simulink library "SG_library"  (R2022b)
settings: Solver=VariableStepAuto  StartTime=0.0  StopTime=10.0  RelTol=1e-3
undefined symbols (not defined in the file or in its folder): a, b, c, dfilt, GeneratorType, IO324, IO324_FPGA, IO324_src, IO334, IO334_FPGA, IO334_src, IO397, IO397_FPGA, IO397_src, repelem
libraries: speedgoatlib_hdlCoder_IO3xx x44, $bdroot x11, slrealtimeutilitieslib x9, simulink x6, hdlsllib x6, dspsrcs4 x2, dsparch4 x2
(part 2 of 3)

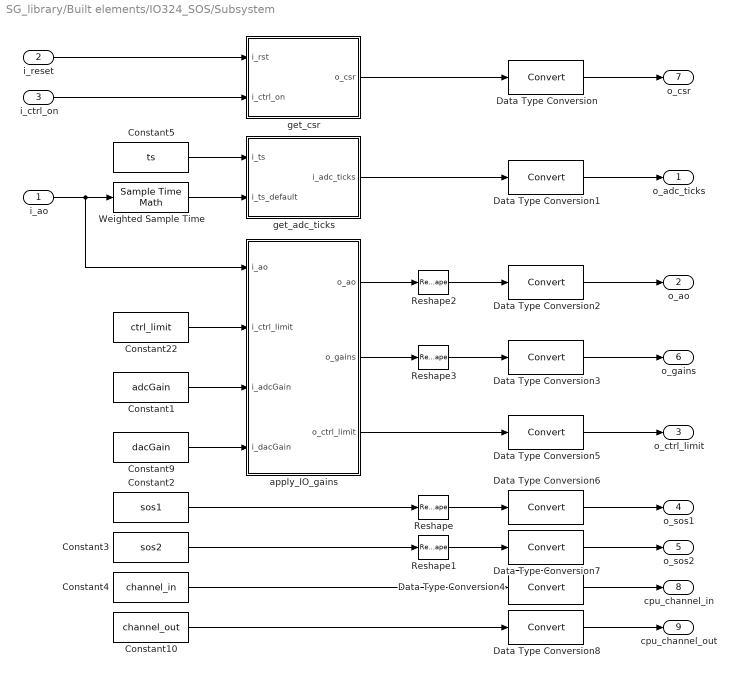
== system SG_library/Built elements/IO324_SOS/Subsystem ==
  i_ao : Inport
  i_reset : Inport  Port=2
  i_ctrl_on : Inport  Port=3
  Constant1 : Constant  Value=adcGain  SampleTime=-1
  Constant10 : Constant  Value=channel_out  SampleTime=-1
  Constant2 : Constant  Value=sos1  SampleTime=-1
  Constant22 : Constant  Value=ctrl_limit  SampleTime=-1
  Constant3 : Constant  Value=sos2  SampleTime=-1
  Constant4 : Constant  Value=channel_in  SampleTime=-1
  Constant5 : Constant  Value=ts  SampleTime=-1
  Constant9 : Constant  Value=dacGain  SampleTime=-1
  Data Type Conversion{,1..8} (9 alike) : DataTypeConversion  SaturateOnIntegerOverflow=off  RndMeth=Floor
  Reshape{,1..3} (4 alike) : Reshape
  Weighted Sample Time : SampleTimeMath  TsampMathOp=Ts Only
  apply_IO_gains : MATLAB Function  TreatAsAtomicUnit=on
  get_adc_ticks : MATLAB Function  TreatAsAtomicUnit=on
  get_csr : MATLAB Function  TreatAsAtomicUnit=on
  o_adc_ticks : Outport
  o_ao : Outport  Port=2
  o_ctrl_limit : Outport  Port=3
  o_sos1 : Outport  Port=4
  o_sos2 : Outport  Port=5
  o_gains : Outport  Port=6
  o_csr : Outport  Port=7
  cpu_channel_in : Outport  Port=8
  cpu_channel_out : Outport  Port=9
  wires:
  i_reset/1 -> get_csr/1(i_rst)
  i_ctrl_on/1 -> get_csr/2(i_ctrl_on)
  Constant5/1 -> get_adc_ticks/1(i_ts)
  Weighted Sample Time/1 -> get_adc_ticks/2(i_ts_default)
  i_ao/1 -> apply_IO_gains/1(i_ao), Weighted Sample Time/1
  get_adc_ticks/1(i_adc_ticks) -> Data Type Conversion1/1
  Constant1/1 -> apply_IO_gains/3(i_adcGain)
  Constant9/1 -> apply_IO_gains/4(i_dacGain)
  Constant22/1 -> apply_IO_gains/2(i_ctrl_limit)
  get_csr/1(o_csr) -> Data Type Conversion/1
  Constant2/1 -> Reshape/1
  Constant3/1 -> Reshape1/1
  Data Type Conversion/1 -> o_csr/1
  Data Type Conversion1/1 -> o_adc_ticks/1
  Data Type Conversion2/1 -> o_ao/1
  Data Type Conversion3/1 -> o_gains/1
  Data Type Conversion5/1 -> o_ctrl_limit/1
  Data Type Conversion6/1 -> o_sos1/1
  Data Type Conversion7/1 -> o_sos2/1
  Reshape/1 -> Data Type Conversion6/1
  Reshape1/1 -> Data Type Conversion7/1
  apply_IO_gains/3(o_ctrl_limit) -> Data Type Conversion5/1
  apply_IO_gains/2(o_gains) -> Reshape3/1
  apply_IO_gains/1(o_ao) -> Reshape2/1
  Reshape2/1 -> Data Type Conversion2/1
  Reshape3/1 -> Data Type Conversion3/1
  Data Type Conversion4/1 -> cpu_channel_in/1
  Constant10/1 -> Data Type Conversion8/1
  Constant4/1 -> Data Type Conversion4/1
  Data Type Conversion8/1 -> cpu_channel_out/1

== system SG_library/Built elements/IO324_SOS/Subsystem1 ==
  i_ai : Inport
  i_ao_monitor : Inport  Port=2
  i_staurated : Inport  Port=3
  Constant1 : Constant  Value=adcGain  SampleTime=-1
  Constant9 : Constant  Value=dacGain  SampleTime=-1
  Data Type Conversion : DataTypeConversion  OutDataTypeStr=double  SaturateOnIntegerOverflow=off  RndMeth=Floor
  Data Type Conversion1 : DataTypeConversion  OutDataTypeStr=double  SaturateOnIntegerOverflow=off  RndMeth=Floor
  Reshape : Reshape
  apply_IO_gains : MATLAB Function  TreatAsAtomicUnit=on
  o_ai : Outport
  o_ao_monitor : Outport  Port=2
  o_saturated : Outport  Port=3
  wires:
  Constant9/1 -> apply_IO_gains/4(i_dacGain)
  apply_IO_gains/1(o_ai) -> Reshape/1
  Constant1/1 -> apply_IO_gains/3(i_adcGain)
  i_ai/1 -> Data Type Conversion/1
  i_ao_monitor/1 -> Data Type Conversion1/1
  Reshape/1 -> o_ai/1
  apply_IO_gains/2(o_ao_monitor) -> o_ao_monitor/1
  Data Type Conversion1/1 -> apply_IO_gains/2(i_ao_monitor)
  Data Type Conversion/1 -> apply_IO_gains/1(i_ai)
  i_staurated/1 -> o_saturated/1

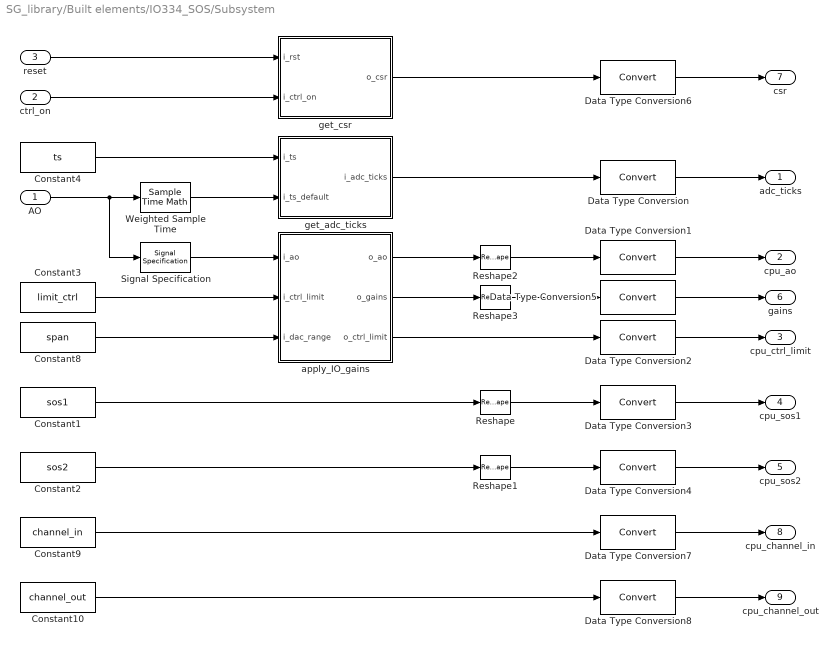
== system SG_library/Built elements/IO334_SOS/Subsystem ==
  AO : Inport
  ctrl_on : Inport  Port=2
  reset : Inport  Port=3
  Constant1 : Constant  Value=sos1  SampleTime=-1
  Constant10 : Constant  Value=channel_out  SampleTime=-1
  Constant2 : Constant  Value=sos2  SampleTime=-1
  Constant3 : Constant  Value=limit_ctrl  SampleTime=-1
  Constant4 : Constant  Value=ts  SampleTime=-1
  Constant8 : Constant  Value=span  SampleTime=-1
  Constant9 : Constant  Value=channel_in  SampleTime=-1
  Data Type Conversion{,1..8} (9 alike) : DataTypeConversion  SaturateOnIntegerOverflow=off  RndMeth=Floor
  Reshape{,1..3} (4 alike) : Reshape
  Signal Specification : SignalSpecification  Dimensions=16
  Weighted Sample Time : SampleTimeMath  TsampMathOp=Ts Only
  apply_IO_gains : MATLAB Function  TreatAsAtomicUnit=on
  get_adc_ticks : MATLAB Function  TreatAsAtomicUnit=on
  get_csr : MATLAB Function  TreatAsAtomicUnit=on
  adc_ticks : Outport
  cpu_ao : Outport  Port=2
  cpu_ctrl_limit : Outport  Port=3
  cpu_sos1 : Outport  Port=4
  cpu_sos2 : Outport  Port=5
  gains : Outport  Port=6
  csr : Outport  Port=7
  cpu_channel_in : Outport  Port=8
  cpu_channel_out : Outport  Port=9
  wires:
  Constant3/1 -> apply_IO_gains/2(i_ctrl_limit)
  apply_IO_gains/1(o_ao) -> Reshape2/1
  apply_IO_gains/3(o_ctrl_limit) -> Data Type Conversion2/1
  apply_IO_gains/2(o_gains) -> Reshape3/1
  get_adc_ticks/1(i_adc_ticks) -> Data Type Conversion/1
  Weighted Sample Time/1 -> get_adc_ticks/2(i_ts_default)
  Constant4/1 -> get_adc_ticks/1(i_ts)
  get_csr/1(o_csr) -> Data Type Conversion6/1
  ctrl_on/1 -> get_csr/2(i_ctrl_on)
  reset/1 -> get_csr/1(i_rst)
  Data Type Conversion6/1 -> csr/1
  Data Type Conversion5/1 -> gains/1
  Data Type Conversion4/1 -> cpu_sos2/1
  Data Type Conversion3/1 -> cpu_sos1/1
  Data Type Conversion2/1 -> cpu_ctrl_limit/1
  Data Type Conversion1/1 -> cpu_ao/1
  Data Type Conversion/1 -> adc_ticks/1
  Reshape1/1 -> Data Type Conversion4/1
  Reshape/1 -> Data Type Conversion3/1
  Constant8/1 -> apply_IO_gains/3(i_dac_range)
  Signal Specification/1 -> apply_IO_gains/1(i_ao)
  Constant1/1 -> Reshape/1
  AO/1 -> Signal Specification/1, Weighted Sample Time/1
  Constant2/1 -> Reshape1/1
  Reshape2/1 -> Data Type Conversion1/1
  Reshape3/1 -> Data Type Conversion5/1
  Constant10/1 -> Data Type Conversion8/1
  Constant9/1 -> Data Type Conversion7/1
  Data Type Conversion7/1 -> cpu_channel_in/1
  Data Type Conversion8/1 -> cpu_channel_out/1

== system SG_library/Built elements/IO334_SOS/Subsystem1 ==
  i_ai : Inport
  i_monitor : Inport  Port=2
  i_staurated : Inport  Port=3
  Constant : Constant  Value=span  SampleTime=-1
  Data Type Conversion : DataTypeConversion  OutDataTypeStr=double  SaturateOnIntegerOverflow=off  RndMeth=Floor
  Data Type Conversion1 : DataTypeConversion  OutDataTypeStr=double  SaturateOnIntegerOverflow=off  RndMeth=Floor
  Reshape : Reshape
  apply_IO_gains : MATLAB Function  TreatAsAtomicUnit=on
  o_ai : Outport
  o_monitor : Outport  Port=2
  o_saturated : Outport  Port=3
  wires:
  apply_IO_gains/1(o_ai) -> Reshape/1
  Constant/1 -> apply_IO_gains/3(i_dac_span)
  i_ai/1 -> Data Type Conversion/1
  i_monitor/1 -> Data Type Conversion1/1
  Reshape/1 -> o_ai/1
  apply_IO_gains/2(o_ao_monitor) -> o_monitor/1
  Data Type Conversion/1 -> apply_IO_gains/1(i_ai)
  Data Type Conversion1/1 -> apply_IO_gains/2(i_ao_monitor)
  i_staurated/1 -> o_saturated/1

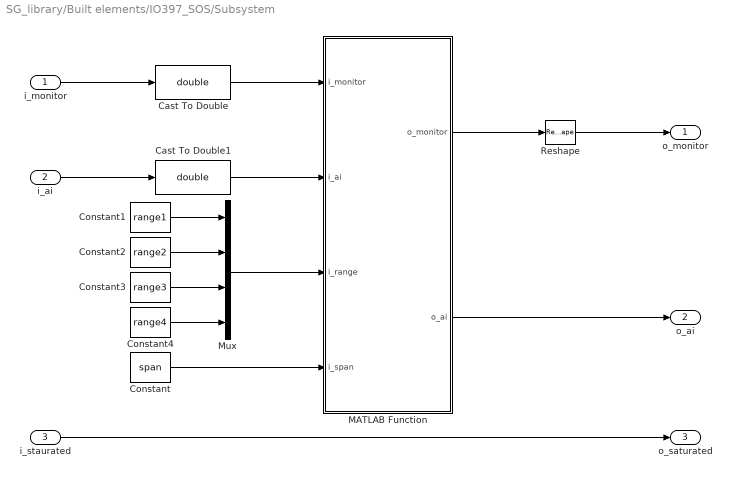
== system SG_library/Built elements/IO397_SOS/Subsystem ==
  i_monitor : Inport
  i_ai : Inport  Port=2
  i_staurated : Inport  Port=3
  Cast To Double : DataTypeConversion  OutDataTypeStr=double  SaturateOnIntegerOverflow=off  RndMeth=Floor
  Cast To Double1 : DataTypeConversion  OutDataTypeStr=double  SaturateOnIntegerOverflow=off  RndMeth=Floor
  Constant : Constant  Value=span  SampleTime=-1
  Constant1 : Constant  Value=range1  SampleTime=-1
  Constant2 : Constant  Value=range2  SampleTime=-1
  Constant3 : Constant  Value=range3  SampleTime=-1
  Constant4 : Constant  Value=range4  SampleTime=-1
  MATLAB Function : MATLAB Function  TreatAsAtomicUnit=on
  Mux : Mux
  Reshape : Reshape
  o_monitor : Outport
  o_ai : Outport  Port=2
  o_saturated : Outport  Port=3
  wires:
  Constant3/1 -> Mux/3
  Constant1/1 -> Mux/1
  MATLAB Function/1(o_monitor) -> Reshape/1
  Constant/1 -> MATLAB Function/4(i_span)
  Constant2/1 -> Mux/2
  Mux/1 -> MATLAB Function/3(i_range)
  Constant4/1 -> Mux/4
  MATLAB Function/2(o_ai) -> o_ai/1
  i_monitor/1 -> Cast To Double/1
  i_ai/1 -> Cast To Double1/1
  Reshape/1 -> o_monitor/1
  Cast To Double/1 -> MATLAB Function/1(i_monitor)
  Cast To Double1/1 -> MATLAB Function/2(i_ai)
  i_staurated/1 -> o_saturated/1

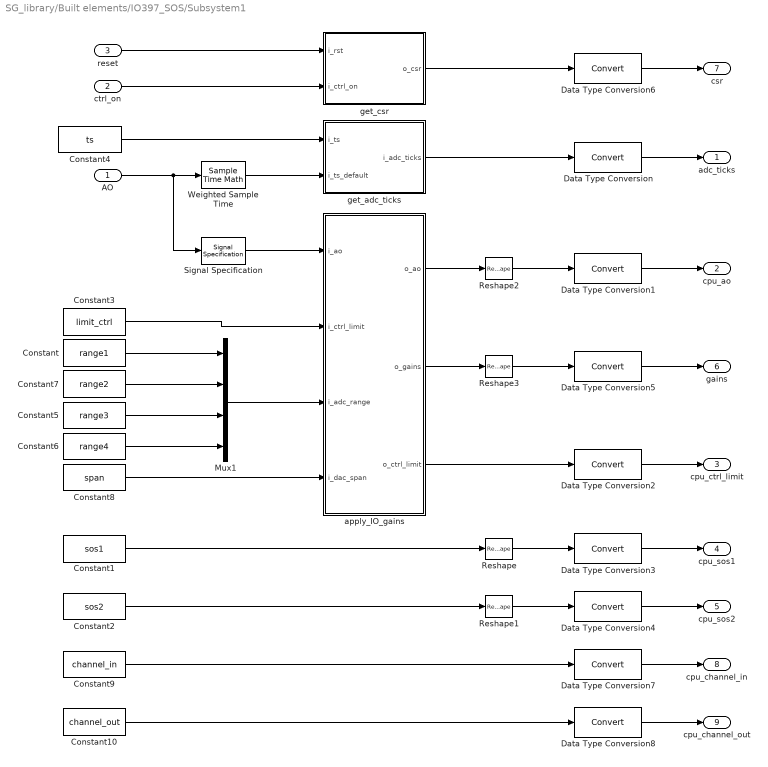
== system SG_library/Built elements/IO397_SOS/Subsystem1 ==
  AO : Inport
  ctrl_on : Inport  Port=2
  reset : Inport  Port=3
  Constant : Constant  Value=range1  SampleTime=-1
  Constant1 : Constant  Value=sos1  SampleTime=-1
  Constant10 : Constant  Value=channel_out  SampleTime=-1
  Constant2 : Constant  Value=sos2  SampleTime=-1
  Constant3 : Constant  Value=limit_ctrl  SampleTime=-1
  Constant4 : Constant  Value=ts  SampleTime=-1
  Constant5 : Constant  Value=range3  SampleTime=-1
  Constant6 : Constant  Value=range4  SampleTime=-1
  Constant7 : Constant  Value=range2  SampleTime=-1
  Constant8 : Constant  Value=span  SampleTime=-1
  Constant9 : Constant  Value=channel_in  SampleTime=-1
  Data Type Conversion{,1..8} (9 alike) : DataTypeConversion  SaturateOnIntegerOverflow=off  RndMeth=Floor
  Mux1 : Mux
  Reshape{,1..3} (4 alike) : Reshape
  Signal Specification : SignalSpecification  Dimensions=4
  Weighted Sample Time : SampleTimeMath  TsampMathOp=Ts Only
  apply_IO_gains : MATLAB Function  TreatAsAtomicUnit=on
  get_adc_ticks : MATLAB Function  TreatAsAtomicUnit=on
  get_csr : MATLAB Function  TreatAsAtomicUnit=on
  adc_ticks : Outport
  cpu_ao : Outport  Port=2
  cpu_ctrl_limit : Outport  Port=3
  cpu_sos1 : Outport  Port=4
  cpu_sos2 : Outport  Port=5
  gains : Outport  Port=6
  csr : Outport  Port=7
  cpu_channel_in : Outport  Port=8
  cpu_channel_out : Outport  Port=9
  wires:
  Constant2/1 -> Reshape1/1
  AO/1 -> Weighted Sample Time/1, Signal Specification/1
  Constant1/1 -> Reshape/1
  Constant7/1 -> Mux1/2
  Signal Specification/1 -> apply_IO_gains/1(i_ao)
  Constant/1 -> Mux1/1
  Mux1/1 -> apply_IO_gains/3(i_adc_range)
  Constant5/1 -> Mux1/3
  Constant6/1 -> Mux1/4
  Constant8/1 -> apply_IO_gains/4(i_dac_span)
  Reshape/1 -> Data Type Conversion3/1
  Reshape1/1 -> Data Type Conversion4/1
  Data Type Conversion/1 -> adc_ticks/1
  Data Type Conversion1/1 -> cpu_ao/1
  Data Type Conversion2/1 -> cpu_ctrl_limit/1
  Data Type Conversion3/1 -> cpu_sos1/1
  Data Type Conversion4/1 -> cpu_sos2/1
  Data Type Conversion5/1 -> gains/1
  Data Type Conversion6/1 -> csr/1
  reset/1 -> get_csr/1(i_rst)
  ctrl_on/1 -> get_csr/2(i_ctrl_on)
  get_csr/1(o_csr) -> Data Type Conversion6/1
  Constant4/1 -> get_adc_ticks/1(i_ts)
  Weighted Sample Time/1 -> get_adc_ticks/2(i_ts_default)
  get_adc_ticks/1(i_adc_ticks) -> Data Type Conversion/1
  apply_IO_gains/2(o_gains) -> Reshape3/1
  apply_IO_gains/1(o_ao) -> Reshape2/1
  Constant3/1 -> apply_IO_gains/2(i_ctrl_limit)
  Reshape2/1 -> Data Type Conversion1/1
  Reshape3/1 -> Data Type Conversion5/1
  apply_IO_gains/3(o_ctrl_limit) -> Data Type Conversion2/1
  Data Type Conversion7/1 -> cpu_channel_in/1
  Data Type Conversion8/1 -> cpu_channel_out/1
  Constant9/1 -> Data Type Conversion7/1
  Constant10/1 -> Data Type Conversion8/1

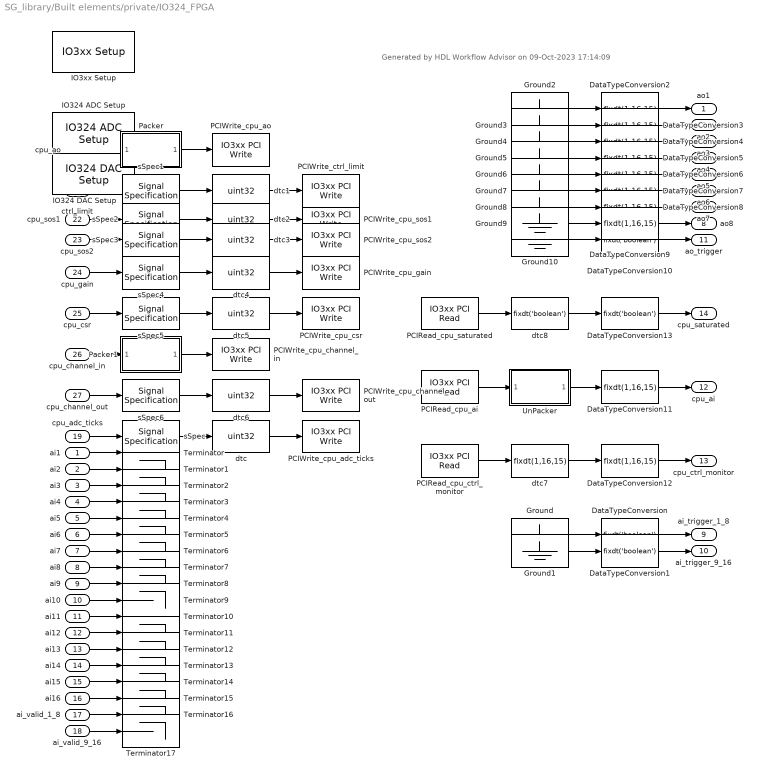
== system SG_library/Built elements/private/IO324_FPGA ==
  note: Generated by HDL Workflow Advisor on 09-Oct-2023 17:14:09
  ai1 : Inport  OutDataTypeStr=fixdt(1,16,15)
  ai2 : Inport  Port=2  OutDataTypeStr=fixdt(1,16,15)
  ai3 : Inport  Port=3  OutDataTypeStr=fixdt(1,16,15)
  ai4 : Inport  Port=4  OutDataTypeStr=fixdt(1,16,15)
  ai5 : Inport  Port=5  OutDataTypeStr=fixdt(1,16,15)
  ai6 : Inport  Port=6  OutDataTypeStr=fixdt(1,16,15)
  ai7 : Inport  Port=7  OutDataTypeStr=fixdt(1,16,15)
  ai8 : Inport  Port=8  OutDataTypeStr=fixdt(1,16,15)
  ai9 : Inport  Port=9  OutDataTypeStr=fixdt(1,16,15)
  ai10 : Inport  Port=10  OutDataTypeStr=fixdt(1,16,15)
  ai11 : Inport  Port=11  OutDataTypeStr=fixdt(1,16,15)
  ai12 : Inport  Port=12  OutDataTypeStr=fixdt(1,16,15)
  ai13 : Inport  Port=13  OutDataTypeStr=fixdt(1,16,15)
  ai14 : Inport  Port=14  OutDataTypeStr=fixdt(1,16,15)
  ai15 : Inport  Port=15  OutDataTypeStr=fixdt(1,16,15)
  ai16 : Inport  Port=16  OutDataTypeStr=fixdt(1,16,15)
  ai_valid_1_8 : Inport  Port=17  OutDataTypeStr=boolean
  ai_valid_9_16 : Inport  Port=18  OutDataTypeStr=boolean
  cpu_adc_ticks : Inport  Port=19  OutDataTypeStr=uint32
  cpu_ao : Inport  Port=20  OutDataTypeStr=fixdt(1,16,15)
  ctrl_limit : Inport  Port=21  OutDataTypeStr=fixdt(1,16,15)
  cpu_sos1 : Inport  Port=22  OutDataTypeStr=fixdt(1,32,26)
  cpu_sos2 : Inport  Port=23  OutDataTypeStr=fixdt(1,32,26)
  cpu_gain : Inport  Port=24  OutDataTypeStr=fixdt(1,32,16)
  cpu_csr : Inport  Port=25  OutDataTypeStr=uint8
  cpu_channel_in : Inport  Port=26
  cpu_channel_out : Inport  Port=27
  DataTypeConversion{,1,10,13} (4 alike) : DataTypeConversion  OutDataTypeStr=fixdt('boolean')  ConvertRealWorld=Stored Integer (SI)  SaturateOnIntegerOverflow=off  RndMeth=Floor
  DataTypeConversion{2..9,11..12} (10 alike) : DataTypeConversion  OutDataTypeStr=fixdt(1,16,15)  ConvertRealWorld=Stored Integer (SI)  SaturateOnIntegerOverflow=off  RndMeth=Floor
  Ground{,1..10} (11 alike) : Ground
  IO324 ADC Setup : speedgoatlib_hdlCoder_IO3xx/IO324 ADC Setup  module_id=module_id  adcGain_1=10.24V  adcActiv_1=on  adcDiffSelect_1=off  adcGain_2=10.24V  adcActiv_2=on  adcDiffSelect_2=off  adcGain_3=10.24V  adcActiv_3=on  adcDiffSelect_3=off  adcGain_4=10.24V  adcActiv_4=on  adcDiffSelect_4=off  adcGain_5=10.24V  adcActiv_5=on  adcDiffSelect_5=off  adcGain_6=10.24V  adcActiv_6=on  adcDiffSelect_6=off  adcGain_7=10.24V  adcActiv_7=on  adcDiffSelect_7=off  adcGain_8=10.24V  adcActiv_8=on  adcDiffSelect_8=off  adcGain_9=10.24V  adcActiv_9=on  adcDiffSelect_9=off  adcGain_10=10.24V  adcActiv_10=on  adcDiffSelect_10=off  adcGain_11=10.24V  adcActiv_11=on  adcDiffSelect_11=off  adcGain_12=10.24V  adcActiv_12=on  adcDiffSelect_12=off  adcGain_13=10.24V  adcActiv_13=on  adcDiffSelect_13=off  adcGain_14=10.24V  adcActiv_14=on  adcDiffSelect_14=off  adcGain_15=10.24V  adcActiv_15=on  adcDiffSelect_15=off  adcGain_16=10.24V  adcActiv_16=on  adcDiffSelect_16=off  adcGain_17=10.24V  adcActiv_17=off  adcDiffSelect_17=off  adcGain_18=10.24V  adcActiv_18=off  adcDiffSelect_18=off  adcGain_19=10.24V  adcActiv_19=off  adcDiffSelect_19=off  adcGain_20=10.24V  adcActiv_20=off  adcDiffSelect_20=off  adcGain_21=10.24V  adcActiv_21=off  adcDiffSelect_21=off  adcGain_22=10.24V  adcActiv_22=off  adcDiffSelect_22=off  adcGain_23=10.24V  adcActiv_23=off  adcDiffSelect_23=off  adcGain_24=10.24V  adcActiv_24=off  adcDiffSelect_24=off  adcGain_25=10.24V  adcActiv_25=off  adcDiffSelect_25=off  adcGain_26=10.24V  adcActiv_26=off  adcDiffSelect_26=off  adcGain_27=10.24V  adcActiv_27=off  adcDiffSelect_27=off  adcGain_28=10.24V  adcActiv_28=off  adcDiffSelect_28=off  adcGain_29=10.24V  adcActiv_29=off  adcDiffSelect_29=off  adcGain_30=10.24V  adcActiv_30=off  adcDiffSelect_30=off  adcGain_31=10.24V  adcActiv_31=off  adcDiffSelect_31=off  adcGain_32=10.24V  adcActiv_32=off  adcDiffSelect_32=off
  IO324 DAC Setup : speedgoatlib_hdlCoder_IO3xx/IO324 DAC Setup  module_id=module_id  dacGain_1=10.0V  dacActiv_1=on  dacGain_2=10.0V  dacActiv_2=on  dacGain_3=10.0V  dacActiv_3=on  dacGain_4=10.0V  dacActiv_4=on  dacGain_5=10.0V  dacActiv_5=on  dacGain_6=10.0V  dacActiv_6=on  dacGain_7=10.0V  dacActiv_7=on  dacGain_8=10.0V  dacActiv_8=on
  IO3xx Setup : speedgoatlib_hdlCoder_IO3xx/IO3xx Setup  mdl_ss_name=IO324_src/IO324_FPGA  board_type=IO324-200k  fpga_sync_mode=on  reset_mode=on  reset_mode_stop=on  device_id=1  module_id=module_id  pci_slot=slot  fpga_mat_file=C:\Speedgoat\Build\IO324_SOS\hdlsrc\IO324_src\IO324_FPGA.mat  timestamp_mcs=10/09/23 17:11:49  timestamp=2310091624  tsreg=hex2dec('8')  bsf_file=IO324_FPGA_2310091624.mcs  mcs=0  device_tree_overlays=Test.dtbo  init_reg_list=[]
  PCIRead_cpu_ai : speedgoatlib_hdlCoder_IO3xx/IO3xx PCI Read  device_id=1  module_id=module_id  board_type=IO324-200k  port_name=cpu_ai  port_offset=hex2dec('220')  port_type=uint32  port_dim=8  strobe=hex2dec('240')  sample_time=ts
  PCIRead_cpu_ctrl_monitor : speedgoatlib_hdlCoder_IO3xx/IO3xx PCI Read  device_id=1  module_id=module_id  board_type=IO324-200k  port_name=cpu_ctrl_monitor  port_offset=hex2dec('120')  port_type=uint32  port_dim=1  strobe=0  sample_time=ts
  PCIRead_cpu_saturated : speedgoatlib_hdlCoder_IO3xx/IO3xx PCI Read  device_id=1  module_id=module_id  board_type=IO324-200k  port_name=cpu_saturated  port_offset=hex2dec('124')  port_type=uint32  port_dim=1  strobe=0  sample_time=ts
  PCIWrite_cpu_adc_ticks : speedgoatlib_hdlCoder_IO3xx/IO3xx PCI Write  device_id=1  module_id=module_id  board_type=IO324-200k  port_name=cpu_adc_ticks  port_offset=hex2dec('100')  port_type=uint32  port_dim=1  strobe=0  sample_time=ts
  PCIWrite_cpu_ao : speedgoatlib_hdlCoder_IO3xx/IO3xx PCI Write  device_id=1  module_id=module_id  board_type=IO324-200k  port_name=cpu_ao  port_offset=hex2dec('130')  port_type=uint32  port_dim=4  strobe=hex2dec('140')  sample_time=ts
  PCIWrite_cpu_channel_in : speedgoatlib_hdlCoder_IO3xx/IO3xx PCI Write  device_id=1  module_id=module_id  board_type=IO324-200k  port_name=cpu_channel_in  port_offset=hex2dec('118')  port_type=uint32  port_dim=1  strobe=0  sample_time=ts
  PCIWrite_cpu_channel_out : speedgoatlib_hdlCoder_IO3xx/IO3xx PCI Write  device_id=1  module_id=module_id  board_type=IO324-200k  port_name=cpu_channel_out  port_offset=hex2dec('11C')  port_type=uint32  port_dim=1  strobe=0  sample_time=ts
  PCIWrite_cpu_csr : speedgoatlib_hdlCoder_IO3xx/IO3xx PCI Write  device_id=1  module_id=module_id  board_type=IO324-200k  port_name=cpu_csr  port_offset=hex2dec('114')  port_type=uint32  port_dim=1  strobe=0  sample_time=ts
  PCIWrite_cpu_gain : speedgoatlib_hdlCoder_IO3xx/IO3xx PCI Write  device_id=1  module_id=module_id  board_type=IO324-200k  port_name=cpu_gain  port_offset=hex2dec('108')  port_type=uint32  port_dim=2  strobe=hex2dec('110')  sample_time=ts
  PCIWrite_cpu_sos1 : speedgoatlib_hdlCoder_IO3xx/IO3xx PCI Write  device_id=1  module_id=module_id  board_type=IO324-200k  port_name=cpu_sos1  port_offset=hex2dec('180')  port_type=uint32  port_dim=24  strobe=hex2dec('200')  sample_time=ts
  PCIWrite_cpu_sos2 : speedgoatlib_hdlCoder_IO3xx/IO3xx PCI Write  device_id=1  module_id=module_id  board_type=IO324-200k  port_name=cpu_sos2  port_offset=hex2dec('280')  port_type=uint32  port_dim=24  strobe=hex2dec('300')  sample_time=ts
  PCIWrite_ctrl_limit : speedgoatlib_hdlCoder_IO3xx/IO3xx PCI Write  device_id=1  module_id=module_id  board_type=IO324-200k  port_name=ctrl_limit  port_offset=hex2dec('104')  port_type=uint32  port_dim=1  strobe=0  sample_time=ts
  Packer : Subsystem
  Packer1 : Subsystem
  Terminator{,1..17} (18 alike) : Terminator
  UnPacker : Subsystem
  dtc{,1..6} (7 alike) : DataTypeConversion  OutDataTypeStr=uint32  ConvertRealWorld=Stored Integer (SI)  SaturateOnIntegerOverflow=off
  dtc7 : DataTypeConversion  OutDataTypeStr=fixdt(1,16,15)  ConvertRealWorld=Stored Integer (SI)  SaturateOnIntegerOverflow=off
  dtc8 : DataTypeConversion  OutDataTypeStr=fixdt('boolean')  ConvertRealWorld=Stored Integer (SI)  SaturateOnIntegerOverflow=off
  sSpec : SignalSpecification  OutDataTypeStr=fixdt(0,32,0)
  sSpec1 : SignalSpecification  OutDataTypeStr=fixdt(1,16,15)
  sSpec2 : SignalSpecification  OutDataTypeStr=fixdt(1,32,26)
  sSpec3 : SignalSpecification  OutDataTypeStr=fixdt(1,32,26)
  sSpec4 : SignalSpecification  OutDataTypeStr=fixdt(1,32,16)
  sSpec5 : SignalSpecification  OutDataTypeStr=fixdt(0,8,0)
  sSpec6 : SignalSpecification  OutDataTypeStr=fixdt(0,8,0)
  ao1 : Outport  VectorParamsAs1DForOutWhenUnconnected=off
  ao2 : Outport  Port=2  VectorParamsAs1DForOutWhenUnconnected=off
  ao3 : Outport  Port=3  VectorParamsAs1DForOutWhenUnconnected=off
  ao4 : Outport  Port=4  VectorParamsAs1DForOutWhenUnconnected=off
  ao5 : Outport  Port=5  VectorParamsAs1DForOutWhenUnconnected=off
  ao6 : Outport  Port=6  VectorParamsAs1DForOutWhenUnconnected=off
  ao7 : Outport  Port=7  VectorParamsAs1DForOutWhenUnconnected=off
  ao8 : Outport  Port=8  VectorParamsAs1DForOutWhenUnconnected=off
  ai_trigger_1_8 : Outport  Port=9  VectorParamsAs1DForOutWhenUnconnected=off
  ai_trigger_9_16 : Outport  Port=10  VectorParamsAs1DForOutWhenUnconnected=off
  ao_trigger : Outport  Port=11  VectorParamsAs1DForOutWhenUnconnected=off
  cpu_ai : Outport  Port=12  VectorParamsAs1DForOutWhenUnconnected=off
  cpu_ctrl_monitor : Outport  Port=13  VectorParamsAs1DForOutWhenUnconnected=off
  cpu_saturated : Outport  Port=14
  wires:
  PCIRead_cpu_saturated/1 -> dtc8/1
  dtc8/1 -> DataTypeConversion13/1
  DataTypeConversion13/1 -> cpu_saturated/1
  PCIRead_cpu_ctrl_monitor/1 -> dtc7/1
  dtc7/1 -> DataTypeConversion12/1
  DataTypeConversion12/1 -> cpu_ctrl_monitor/1
  PCIRead_cpu_ai/1 -> UnPacker/1(packed)
  UnPacker/1(unpacked) -> DataTypeConversion11/1
  DataTypeConversion11/1 -> cpu_ai/1
  dtc6/1 -> PCIWrite_cpu_channel_out/1
  sSpec6/1 -> dtc6/1
  cpu_channel_out/1 -> sSpec6/1
  Packer1/1(packed) -> PCIWrite_cpu_channel_in/1
  cpu_channel_in/1 -> Packer1/1(unpacked)
  dtc5/1 -> PCIWrite_cpu_csr/1
  sSpec5/1 -> dtc5/1
  cpu_csr/1 -> sSpec5/1
  dtc4/1 -> PCIWrite_cpu_gain/1
  sSpec4/1 -> dtc4/1
  cpu_gain/1 -> sSpec4/1
  dtc3/1 -> PCIWrite_cpu_sos2/1
  sSpec3/1 -> dtc3/1
  cpu_sos2/1 -> sSpec3/1
  dtc2/1 -> PCIWrite_cpu_sos1/1
  sSpec2/1 -> dtc2/1
  cpu_sos1/1 -> sSpec2/1
  dtc1/1 -> PCIWrite_ctrl_limit/1
  sSpec1/1 -> dtc1/1
  ctrl_limit/1 -> sSpec1/1
  Packer/1(packed) -> PCIWrite_cpu_ao/1
  cpu_ao/1 -> Packer/1(unpacked)
  dtc/1 -> PCIWrite_cpu_adc_ticks/1
  sSpec/1 -> dtc/1
  cpu_adc_ticks/1 -> sSpec/1
  Ground10/1 -> DataTypeConversion10/1
  DataTypeConversion10/1 -> ao_trigger/1
  Ground9/1 -> DataTypeConversion9/1
  DataTypeConversion9/1 -> ao8/1
  Ground8/1 -> DataTypeConversion8/1
  DataTypeConversion8/1 -> ao7/1
  Ground7/1 -> DataTypeConversion7/1
  DataTypeConversion7/1 -> ao6/1
  Ground6/1 -> DataTypeConversion6/1
  DataTypeConversion6/1 -> ao5/1
  Ground5/1 -> DataTypeConversion5/1
  DataTypeConversion5/1 -> ao4/1
  Ground4/1 -> DataTypeConversion4/1
  DataTypeConversion4/1 -> ao3/1
  Ground3/1 -> DataTypeConversion3/1
  DataTypeConversion3/1 -> ao2/1
  Ground2/1 -> DataTypeConversion2/1
  DataTypeConversion2/1 -> ao1/1
  Ground1/1 -> DataTypeConversion1/1
  DataTypeConversion1/1 -> ai_trigger_9_16/1
  Ground/1 -> DataTypeConversion/1
  DataTypeConversion/1 -> ai_trigger_1_8/1
  ai_valid_9_16/1 -> Terminator17/1
  ai_valid_1_8/1 -> Terminator16/1
  ai16/1 -> Terminator15/1
  ai15/1 -> Terminator14/1
  ai14/1 -> Terminator13/1
  ai13/1 -> Terminator12/1
  ai12/1 -> Terminator11/1
  ai11/1 -> Terminator10/1
  ai10/1 -> Terminator9/1
  ai9/1 -> Terminator8/1
  ai8/1 -> Terminator7/1
  ai7/1 -> Terminator6/1
  ai6/1 -> Terminator5/1
  ai5/1 -> Terminator4/1
  ai4/1 -> Terminator3/1
  ai3/1 -> Terminator2/1
  ai2/1 -> Terminator1/1
  ai1/1 -> Terminator/1

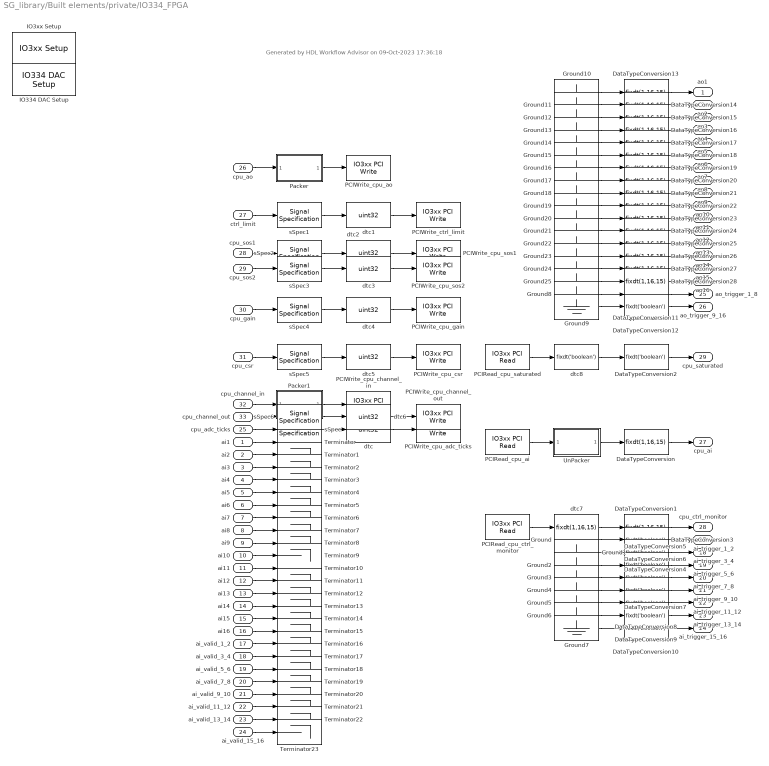
== system SG_library/Built elements/private/IO334_FPGA ==
  note: Generated by HDL Workflow Advisor on 09-Oct-2023 17:36:18
  ai1 : Inport  OutDataTypeStr=fixdt(1,16,15)
  ai2 : Inport  Port=2  OutDataTypeStr=fixdt(1,16,15)
  ai3 : Inport  Port=3  OutDataTypeStr=fixdt(1,16,15)
  ai4 : Inport  Port=4  OutDataTypeStr=fixdt(1,16,15)
  ai5 : Inport  Port=5  OutDataTypeStr=fixdt(1,16,15)
  ai6 : Inport  Port=6  OutDataTypeStr=fixdt(1,16,15)
  ai7 : Inport  Port=7  OutDataTypeStr=fixdt(1,16,15)
  ai8 : Inport  Port=8  OutDataTypeStr=fixdt(1,16,15)
  ai9 : Inport  Port=9  OutDataTypeStr=fixdt(1,16,15)
  ai10 : Inport  Port=10  OutDataTypeStr=fixdt(1,16,15)
  ai11 : Inport  Port=11  OutDataTypeStr=fixdt(1,16,15)
  ai12 : Inport  Port=12  OutDataTypeStr=fixdt(1,16,15)
  ai13 : Inport  Port=13  OutDataTypeStr=fixdt(1,16,15)
  ai14 : Inport  Port=14  OutDataTypeStr=fixdt(1,16,15)
  ai15 : Inport  Port=15  OutDataTypeStr=fixdt(1,16,15)
  ai16 : Inport  Port=16  OutDataTypeStr=fixdt(1,16,15)
  ai_valid_1_2 : Inport  Port=17  OutDataTypeStr=boolean
  ai_valid_3_4 : Inport  Port=18  OutDataTypeStr=boolean
  ai_valid_5_6 : Inport  Port=19  OutDataTypeStr=boolean
  ai_valid_7_8 : Inport  Port=20  OutDataTypeStr=boolean
  ai_valid_9_10 : Inport  Port=21  OutDataTypeStr=boolean
  ai_valid_11_12 : Inport  Port=22  OutDataTypeStr=boolean
  ai_valid_13_14 : Inport  Port=23  OutDataTypeStr=boolean
  ai_valid_15_16 : Inport  Port=24  OutDataTypeStr=boolean
  cpu_adc_ticks : Inport  Port=25  OutDataTypeStr=uint32
  cpu_ao : Inport  Port=26  OutDataTypeStr=fixdt(1,16,15)
  ctrl_limit : Inport  Port=27  OutDataTypeStr=fixdt(1,16,15)
  cpu_sos1 : Inport  Port=28  OutDataTypeStr=fixdt(1,32,26)
  cpu_sos2 : Inport  Port=29  OutDataTypeStr=fixdt(1,32,26)
  cpu_gain : Inport  Port=30  OutDataTypeStr=fixdt(1,32,16)
  cpu_csr : Inport  Port=31  OutDataTypeStr=uint8
  cpu_channel_in : Inport  Port=32
  cpu_channel_out : Inport  Port=33
  DataTypeConversion{,1,13..28} (18 alike) : DataTypeConversion  OutDataTypeStr=fixdt(1,16,15)  ConvertRealWorld=Stored Integer (SI)  SaturateOnIntegerOverflow=off  RndMeth=Floor
  DataTypeConversion{2..12} (11 alike) : DataTypeConversion  OutDataTypeStr=fixdt('boolean')  ConvertRealWorld=Stored Integer (SI)  SaturateOnIntegerOverflow=off  RndMeth=Floor
  Ground{,1..25} (26 alike) : Ground
  IO334 DAC Setup : speedgoatlib_hdlCoder_IO3xx/IO334 DAC Setup  module_id=module_id  OutputRange=Auto (same as ADC)
  IO3xx Setup : speedgoatlib_hdlCoder_IO3xx/IO3xx Setup  mdl_ss_name=IO334_src/IO334_FPGA  board_type=IO334-325k  fpga_sync_mode=on  reset_mode=on  reset_mode_stop=on  device_id=1  module_id=module_id  pci_slot=slot  fpga_mat_file=C:\Speedgoat\Build\IO334_SOS\hdlsrc\IO334_src\IO334_FPGA.mat  timestamp_mcs=10/09/23 17:33:47  timestamp=2310091715  tsreg=hex2dec('8')  bsf_file=IO334_FPGA_2310091715.mcs  mcs=0  device_tree_overlays=Test.dtbo  init_reg_list=[]
  PCIRead_cpu_ai : speedgoatlib_hdlCoder_IO3xx/IO3xx PCI Read  device_id=1  module_id=module_id  board_type=IO334-325k  port_name=cpu_ai  port_offset=hex2dec('220')  port_type=uint32  port_dim=8  strobe=hex2dec('240')  sample_time=ts
  PCIRead_cpu_ctrl_monitor : speedgoatlib_hdlCoder_IO3xx/IO3xx PCI Read  device_id=1  module_id=module_id  board_type=IO334-325k  port_name=cpu_ctrl_monitor  port_offset=hex2dec('120')  port_type=uint32  port_dim=1  strobe=0  sample_time=ts
  PCIRead_cpu_saturated : speedgoatlib_hdlCoder_IO3xx/IO3xx PCI Read  device_id=1  module_id=module_id  board_type=IO334-325k  port_name=cpu_saturated  port_offset=hex2dec('124')  port_type=uint32  port_dim=1  strobe=0  sample_time=ts
  PCIWrite_cpu_adc_ticks : speedgoatlib_hdlCoder_IO3xx/IO3xx PCI Write  device_id=1  module_id=module_id  board_type=IO334-325k  port_name=cpu_adc_ticks  port_offset=hex2dec('100')  port_type=uint32  port_dim=1  strobe=0  sample_time=ts
  PCIWrite_cpu_ao : speedgoatlib_hdlCoder_IO3xx/IO3xx PCI Write  device_id=1  module_id=module_id  board_type=IO334-325k  port_name=cpu_ao  port_offset=hex2dec('140')  port_type=uint32  port_dim=8  strobe=hex2dec('160')  sample_time=ts
  PCIWrite_cpu_channel_in : speedgoatlib_hdlCoder_IO3xx/IO3xx PCI Write  device_id=1  module_id=module_id  board_type=IO334-325k  port_name=cpu_channel_in  port_offset=hex2dec('118')  port_type=uint32  port_dim=1  strobe=0  sample_time=ts
  PCIWrite_cpu_channel_out : speedgoatlib_hdlCoder_IO3xx/IO3xx PCI Write  device_id=1  module_id=module_id  board_type=IO334-325k  port_name=cpu_channel_out  port_offset=hex2dec('11C')  port_type=uint32  port_dim=1  strobe=0  sample_time=ts
  PCIWrite_cpu_csr : speedgoatlib_hdlCoder_IO3xx/IO3xx PCI Write  device_id=1  module_id=module_id  board_type=IO334-325k  port_name=cpu_csr  port_offset=hex2dec('114')  port_type=uint32  port_dim=1  strobe=0  sample_time=ts
  PCIWrite_cpu_gain : speedgoatlib_hdlCoder_IO3xx/IO3xx PCI Write  device_id=1  module_id=module_id  board_type=IO334-325k  port_name=cpu_gain  port_offset=hex2dec('108')  port_type=uint32  port_dim=2  strobe=hex2dec('110')  sample_time=ts
  PCIWrite_cpu_sos1 : speedgoatlib_hdlCoder_IO3xx/IO3xx PCI Write  device_id=1  module_id=module_id  board_type=IO334-325k  port_name=cpu_sos1  port_offset=hex2dec('180')  port_type=uint32  port_dim=24  strobe=hex2dec('200')  sample_time=ts
  PCIWrite_cpu_sos2 : speedgoatlib_hdlCoder_IO3xx/IO3xx PCI Write  device_id=1  module_id=module_id  board_type=IO334-325k  port_name=cpu_sos2  port_offset=hex2dec('280')  port_type=uint32  port_dim=24  strobe=hex2dec('300')  sample_time=ts
  PCIWrite_ctrl_limit : speedgoatlib_hdlCoder_IO3xx/IO3xx PCI Write  device_id=1  module_id=module_id  board_type=IO334-325k  port_name=ctrl_limit  port_offset=hex2dec('104')  port_type=uint32  port_dim=1  strobe=0  sample_time=ts
  Packer : Subsystem
  Packer1 : Subsystem
  Terminator{,1..23} (24 alike) : Terminator
  UnPacker : Subsystem
  dtc{,1..6} (7 alike) : DataTypeConversion  OutDataTypeStr=uint32  ConvertRealWorld=Stored Integer (SI)  SaturateOnIntegerOverflow=off
  dtc7 : DataTypeConversion  OutDataTypeStr=fixdt(1,16,15)  ConvertRealWorld=Stored Integer (SI)  SaturateOnIntegerOverflow=off
  dtc8 : DataTypeConversion  OutDataTypeStr=fixdt('boolean')  ConvertRealWorld=Stored Integer (SI)  SaturateOnIntegerOverflow=off
  sSpec : SignalSpecification  OutDataTypeStr=fixdt(0,32,0)
  sSpec1 : SignalSpecification  OutDataTypeStr=fixdt(1,16,15)
  sSpec2 : SignalSpecification  OutDataTypeStr=fixdt(1,32,26)
  sSpec3 : SignalSpecification  OutDataTypeStr=fixdt(1,32,26)
  sSpec4 : SignalSpecification  OutDataTypeStr=fixdt(1,32,16)
  sSpec5 : SignalSpecification  OutDataTypeStr=fixdt(0,8,0)
  sSpec6 : SignalSpecification  OutDataTypeStr=fixdt(0,8,0)
  ao1 : Outport  VectorParamsAs1DForOutWhenUnconnected=off
  ao2 : Outport  Port=2  VectorParamsAs1DForOutWhenUnconnected=off
  ao3 : Outport  Port=3  VectorParamsAs1DForOutWhenUnconnected=off
  ao4 : Outport  Port=4  VectorParamsAs1DForOutWhenUnconnected=off
  ao5 : Outport  Port=5  VectorParamsAs1DForOutWhenUnconnected=off
  ao6 : Outport  Port=6  VectorParamsAs1DForOutWhenUnconnected=off
  ao7 : Outport  Port=7  VectorParamsAs1DForOutWhenUnconnected=off
  ao8 : Outport  Port=8  VectorParamsAs1DForOutWhenUnconnected=off
  ao9 : Outport  Port=9  VectorParamsAs1DForOutWhenUnconnected=off
  ao10 : Outport  Port=10  VectorParamsAs1DForOutWhenUnconnected=off
  ao11 : Outport  Port=11  VectorParamsAs1DForOutWhenUnconnected=off
  ao12 : Outport  Port=12  VectorParamsAs1DForOutWhenUnconnected=off
  ao13 : Outport  Port=13  VectorParamsAs1DForOutWhenUnconnected=off
  ao14 : Outport  Port=14  VectorParamsAs1DForOutWhenUnconnected=off
  ao15 : Outport  Port=15  VectorParamsAs1DForOutWhenUnconnected=off
  ao16 : Outport  Port=16  VectorParamsAs1DForOutWhenUnconnected=off
  ai_trigger_1_2 : Outport  Port=17  VectorParamsAs1DForOutWhenUnconnected=off
  ai_trigger_3_4 : Outport  Port=18  VectorParamsAs1DForOutWhenUnconnected=off
  ai_trigger_5_6 : Outport  Port=19  VectorParamsAs1DForOutWhenUnconnected=off
  ai_trigger_7_8 : Outport  Port=20  VectorParamsAs1DForOutWhenUnconnected=off
  ai_trigger_9_10 : Outport  Port=21  VectorParamsAs1DForOutWhenUnconnected=off
  ai_trigger_11_12 : Outport  Port=22  VectorParamsAs1DForOutWhenUnconnected=off
  ai_trigger_13_14 : Outport  Port=23  VectorParamsAs1DForOutWhenUnconnected=off
  ai_trigger_15_16 : Outport  Port=24  VectorParamsAs1DForOutWhenUnconnected=off
  ao_trigger_1_8 : Outport  Port=25  VectorParamsAs1DForOutWhenUnconnected=off
  ao_trigger_9_16 : Outport  Port=26  VectorParamsAs1DForOutWhenUnconnected=off
  cpu_ai : Outport  Port=27  VectorParamsAs1DForOutWhenUnconnected=off
  cpu_ctrl_monitor : Outport  Port=28  VectorParamsAs1DForOutWhenUnconnected=off
  cpu_saturated : Outport  Port=29
  wires:
  Ground25/1 -> DataTypeConversion28/1
  DataTypeConversion28/1 -> ao16/1
  Ground24/1 -> DataTypeConversion27/1
  DataTypeConversion27/1 -> ao15/1
  Ground23/1 -> DataTypeConversion26/1
  DataTypeConversion26/1 -> ao14/1
  Ground22/1 -> DataTypeConversion25/1
  DataTypeConversion25/1 -> ao13/1
  Ground21/1 -> DataTypeConversion24/1
  DataTypeConversion24/1 -> ao12/1
  Ground20/1 -> DataTypeConversion23/1
  DataTypeConversion23/1 -> ao11/1
  Ground19/1 -> DataTypeConversion22/1
  DataTypeConversion22/1 -> ao10/1
  Ground18/1 -> DataTypeConversion21/1
  DataTypeConversion21/1 -> ao9/1
  Ground17/1 -> DataTypeConversion20/1
  DataTypeConversion20/1 -> ao8/1
  Ground16/1 -> DataTypeConversion19/1
  DataTypeConversion19/1 -> ao7/1
  Ground15/1 -> DataTypeConversion18/1
  DataTypeConversion18/1 -> ao6/1
  Ground14/1 -> DataTypeConversion17/1
  DataTypeConversion17/1 -> ao5/1
  Ground13/1 -> DataTypeConversion16/1
  DataTypeConversion16/1 -> ao4/1
  Ground12/1 -> DataTypeConversion15/1
  DataTypeConversion15/1 -> ao3/1
  Ground11/1 -> DataTypeConversion14/1
  DataTypeConversion14/1 -> ao2/1
  Ground10/1 -> DataTypeConversion13/1
  DataTypeConversion13/1 -> ao1/1
  Ground9/1 -> DataTypeConversion12/1
  DataTypeConversion12/1 -> ao_trigger_9_16/1
  Ground8/1 -> DataTypeConversion11/1
  DataTypeConversion11/1 -> ao_trigger_1_8/1
  Ground7/1 -> DataTypeConversion10/1
  DataTypeConversion10/1 -> ai_trigger_15_16/1
  Ground6/1 -> DataTypeConversion9/1
  DataTypeConversion9/1 -> ai_trigger_13_14/1
  Ground5/1 -> DataTypeConversion8/1
  DataTypeConversion8/1 -> ai_trigger_11_12/1
  Ground4/1 -> DataTypeConversion7/1
  DataTypeConversion7/1 -> ai_trigger_9_10/1
  Ground3/1 -> DataTypeConversion6/1
  DataTypeConversion6/1 -> ai_trigger_7_8/1
  Ground2/1 -> DataTypeConversion5/1
  DataTypeConversion5/1 -> ai_trigger_5_6/1
  Ground1/1 -> DataTypeConversion4/1
  DataTypeConversion4/1 -> ai_trigger_3_4/1
  Ground/1 -> DataTypeConversion3/1
  DataTypeConversion3/1 -> ai_trigger_1_2/1
  ai_valid_15_16/1 -> Terminator23/1
  ai_valid_13_14/1 -> Terminator22/1
  ai_valid_11_12/1 -> Terminator21/1
  ai_valid_9_10/1 -> Terminator20/1
  ai_valid_7_8/1 -> Terminator19/1
  ai_valid_5_6/1 -> Terminator18/1
  ai_valid_3_4/1 -> Terminator17/1
  ai_valid_1_2/1 -> Terminator16/1
  ai16/1 -> Terminator15/1
  ai15/1 -> Terminator14/1
  ai14/1 -> Terminator13/1
  ai13/1 -> Terminator12/1
  ai12/1 -> Terminator11/1
  ai11/1 -> Terminator10/1
  ai10/1 -> Terminator9/1
  ai9/1 -> Terminator8/1
  ai8/1 -> Terminator7/1
  ai7/1 -> Terminator6/1
  ai6/1 -> Terminator5/1
  ai5/1 -> Terminator4/1
  ai4/1 -> Terminator3/1
  ai3/1 -> Terminator2/1
  ai2/1 -> Terminator1/1
  ai1/1 -> Terminator/1
  PCIRead_cpu_saturated/1 -> dtc8/1
  dtc8/1 -> DataTypeConversion2/1
  DataTypeConversion2/1 -> cpu_saturated/1
  PCIRead_cpu_ctrl_monitor/1 -> dtc7/1
  dtc7/1 -> DataTypeConversion1/1
  DataTypeConversion1/1 -> cpu_ctrl_monitor/1
  PCIRead_cpu_ai/1 -> UnPacker/1(packed)
  UnPacker/1(unpacked) -> DataTypeConversion/1
  DataTypeConversion/1 -> cpu_ai/1
  dtc6/1 -> PCIWrite_cpu_channel_out/1
  sSpec6/1 -> dtc6/1
  cpu_channel_out/1 -> sSpec6/1
  Packer1/1(packed) -> PCIWrite_cpu_channel_in/1
  cpu_channel_in/1 -> Packer1/1(unpacked)
  dtc5/1 -> PCIWrite_cpu_csr/1
  sSpec5/1 -> dtc5/1
  cpu_csr/1 -> sSpec5/1
  dtc4/1 -> PCIWrite_cpu_gain/1
  sSpec4/1 -> dtc4/1
  cpu_gain/1 -> sSpec4/1
  dtc3/1 -> PCIWrite_cpu_sos2/1
  sSpec3/1 -> dtc3/1
  cpu_sos2/1 -> sSpec3/1
  dtc2/1 -> PCIWrite_cpu_sos1/1
  sSpec2/1 -> dtc2/1
  cpu_sos1/1 -> sSpec2/1
  dtc1/1 -> PCIWrite_ctrl_limit/1
  sSpec1/1 -> dtc1/1
  ctrl_limit/1 -> sSpec1/1
  Packer/1(packed) -> PCIWrite_cpu_ao/1
  cpu_ao/1 -> Packer/1(unpacked)
  dtc/1 -> PCIWrite_cpu_adc_ticks/1
  sSpec/1 -> dtc/1
  cpu_adc_ticks/1 -> sSpec/1

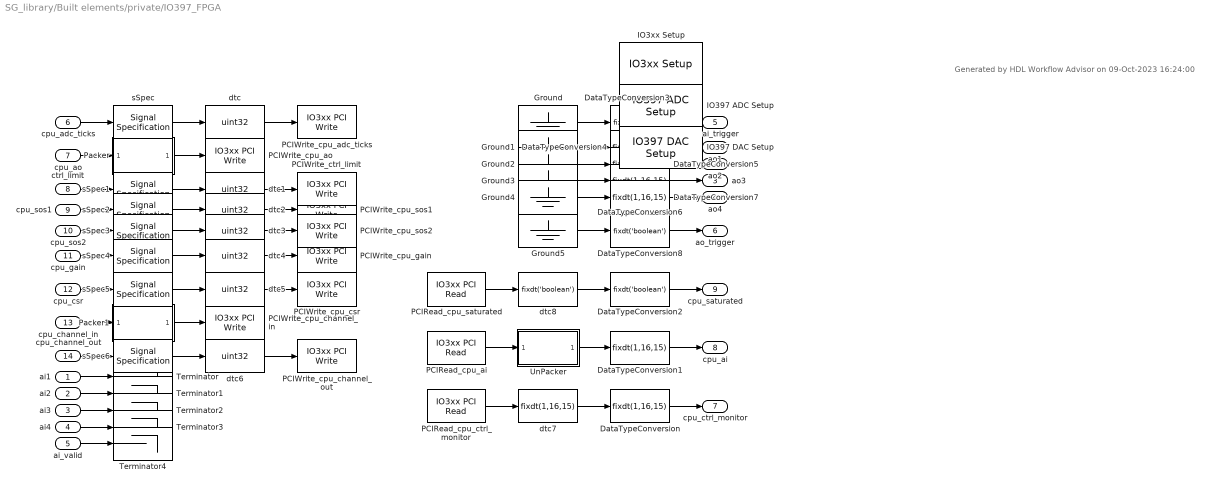
== system SG_library/Built elements/private/IO397_FPGA ==
  note: Generated by HDL Workflow Advisor on 09-Oct-2023 16:24:00
  ai1 : Inport  OutDataTypeStr=fixdt(1,16,15)
  ai2 : Inport  Port=2  OutDataTypeStr=fixdt(1,16,15)
  ai3 : Inport  Port=3  OutDataTypeStr=fixdt(1,16,15)
  ai4 : Inport  Port=4  OutDataTypeStr=fixdt(1,16,15)
  ai_valid : Inport  Port=5  OutDataTypeStr=boolean
  cpu_adc_ticks : Inport  Port=6  OutDataTypeStr=uint32
  cpu_ao : Inport  Port=7  OutDataTypeStr=fixdt(1,16,15)
  ctrl_limit : Inport  Port=8  OutDataTypeStr=fixdt(1,16,15)
  cpu_sos1 : Inport  Port=9  OutDataTypeStr=fixdt(1,32,26)
  cpu_sos2 : Inport  Port=10  OutDataTypeStr=fixdt(1,32,26)
  cpu_gain : Inport  Port=11  OutDataTypeStr=fixdt(1,32,16)
  cpu_csr : Inport  Port=12  OutDataTypeStr=uint8
  cpu_channel_in : Inport  Port=13
  cpu_channel_out : Inport  Port=14
  DataTypeConversion{,1,4..7} (6 alike) : DataTypeConversion  OutDataTypeStr=fixdt(1,16,15)  ConvertRealWorld=Stored Integer (SI)  SaturateOnIntegerOverflow=off  RndMeth=Floor
  DataTypeConversion2 : DataTypeConversion  OutDataTypeStr=fixdt('boolean')  ConvertRealWorld=Stored Integer (SI)  SaturateOnIntegerOverflow=off  RndMeth=Floor
  DataTypeConversion3 : DataTypeConversion  OutDataTypeStr=fixdt('boolean')  ConvertRealWorld=Stored Integer (SI)  SaturateOnIntegerOverflow=off  RndMeth=Floor
  DataTypeConversion8 : DataTypeConversion  OutDataTypeStr=fixdt('boolean')  ConvertRealWorld=Stored Integer (SI)  SaturateOnIntegerOverflow=off  RndMeth=Floor
  Ground{,1..5} (6 alike) : Ground
  IO397 ADC Setup : speedgoatlib_hdlCoder_IO3xx/IO397 ADC Setup  module_id=module_id  range1=+-10 V  range2=+-10 V  range3=+-10 V  range4=+-10 V
  IO397 DAC Setup : speedgoatlib_hdlCoder_IO3xx/IO397 DAC Setup  module_id=module_id  span=+-10 V
  IO3xx Setup : speedgoatlib_hdlCoder_IO3xx/IO3xx Setup  mdl_ss_name=IO397_src/IO397_FPGA  board_type=IO397-50k  fpga_sync_mode=on  reset_mode=on  reset_mode_stop=on  device_id=1  module_id=module_id  pci_slot=slot  fpga_mat_file=C:\Speedgoat\Build\IO397_SOS\hdlsrc\IO397_src\IO397_FPGA.mat  timestamp_mcs=10/09/23 16:22:53  timestamp=2310091612  tsreg=hex2dec('8')  bsf_file=IO397_FPGA_2310091612.mcs  mcs=0  device_tree_overlays=Test.dtbo  init_reg_list=[]
  PCIRead_cpu_ai : speedgoatlib_hdlCoder_IO3xx/IO3xx PCI Read  device_id=1  module_id=module_id  board_type=IO397-50k  port_name=cpu_ai  port_offset=hex2dec('120')  port_type=uint32  port_dim=2  strobe=hex2dec('128')  sample_time=ts
  PCIRead_cpu_ctrl_monitor : speedgoatlib_hdlCoder_IO3xx/IO3xx PCI Read  device_id=1  module_id=module_id  board_type=IO397-50k  port_name=cpu_ctrl_monitor  port_offset=hex2dec('13C')  port_type=uint32  port_dim=1  strobe=0  sample_time=ts
  PCIRead_cpu_saturated : speedgoatlib_hdlCoder_IO3xx/IO3xx PCI Read  device_id=1  module_id=module_id  board_type=IO397-50k  port_name=cpu_saturated  port_offset=hex2dec('12C')  port_type=uint32  port_dim=1  strobe=0  sample_time=ts
  PCIWrite_cpu_adc_ticks : speedgoatlib_hdlCoder_IO3xx/IO3xx PCI Write  device_id=1  module_id=module_id  board_type=IO397-50k  port_name=cpu_adc_ticks  port_offset=hex2dec('100')  port_type=uint32  port_dim=1  strobe=0  sample_time=ts
  PCIWrite_cpu_ao : speedgoatlib_hdlCoder_IO3xx/IO3xx PCI Write  device_id=1  module_id=module_id  board_type=IO397-50k  port_name=cpu_ao  port_offset=hex2dec('130')  port_type=uint32  port_dim=2  strobe=hex2dec('138')  sample_time=ts
  PCIWrite_cpu_channel_in : speedgoatlib_hdlCoder_IO3xx/IO3xx PCI Write  device_id=1  module_id=module_id  board_type=IO397-50k  port_name=cpu_channel_in  port_offset=hex2dec('118')  port_type=uint32  port_dim=1  strobe=0  sample_time=ts
  PCIWrite_cpu_channel_out : speedgoatlib_hdlCoder_IO3xx/IO3xx PCI Write  device_id=1  module_id=module_id  board_type=IO397-50k  port_name=cpu_channel_out  port_offset=hex2dec('11C')  port_type=uint32  port_dim=1  strobe=0  sample_time=ts
  PCIWrite_cpu_csr : speedgoatlib_hdlCoder_IO3xx/IO3xx PCI Write  device_id=1  module_id=module_id  board_type=IO397-50k  port_name=cpu_csr  port_offset=hex2dec('114')  port_type=uint32  port_dim=1  strobe=0  sample_time=ts
  PCIWrite_cpu_gain : speedgoatlib_hdlCoder_IO3xx/IO3xx PCI Write  device_id=1  module_id=module_id  board_type=IO397-50k  port_name=cpu_gain  port_offset=hex2dec('108')  port_type=uint32  port_dim=2  strobe=hex2dec('110')  sample_time=ts
  PCIWrite_cpu_sos1 : speedgoatlib_hdlCoder_IO3xx/IO3xx PCI Write  device_id=1  module_id=module_id  board_type=IO397-50k  port_name=cpu_sos1  port_offset=hex2dec('180')  port_type=uint32  port_dim=24  strobe=hex2dec('200')  sample_time=ts
  PCIWrite_cpu_sos2 : speedgoatlib_hdlCoder_IO3xx/IO3xx PCI Write  device_id=1  module_id=module_id  board_type=IO397-50k  port_name=cpu_sos2  port_offset=hex2dec('280')  port_type=uint32  port_dim=24  strobe=hex2dec('300')  sample_time=ts
  PCIWrite_ctrl_limit : speedgoatlib_hdlCoder_IO3xx/IO3xx PCI Write  device_id=1  module_id=module_id  board_type=IO397-50k  port_name=ctrl_limit  port_offset=hex2dec('104')  port_type=uint32  port_dim=1  strobe=0  sample_time=ts
  Packer : Subsystem
  Packer1 : Subsystem
  Terminator{,1..4} (5 alike) : Terminator
  UnPacker : Subsystem
  dtc{,1..6} (7 alike) : DataTypeConversion  OutDataTypeStr=uint32  ConvertRealWorld=Stored Integer (SI)  SaturateOnIntegerOverflow=off
  dtc7 : DataTypeConversion  OutDataTypeStr=fixdt(1,16,15)  ConvertRealWorld=Stored Integer (SI)  SaturateOnIntegerOverflow=off
  dtc8 : DataTypeConversion  OutDataTypeStr=fixdt('boolean')  ConvertRealWorld=Stored Integer (SI)  SaturateOnIntegerOverflow=off
  sSpec : SignalSpecification  OutDataTypeStr=fixdt(0,32,0)
  sSpec1 : SignalSpecification  OutDataTypeStr=fixdt(1,16,15)
  sSpec2 : SignalSpecification  OutDataTypeStr=fixdt(1,32,26)
  sSpec3 : SignalSpecification  OutDataTypeStr=fixdt(1,32,26)
  sSpec4 : SignalSpecification  OutDataTypeStr=fixdt(1,32,16)
  sSpec5 : SignalSpecification  OutDataTypeStr=fixdt(0,8,0)
  sSpec6 : SignalSpecification  OutDataTypeStr=fixdt(0,8,0)
  ao1 : Outport  VectorParamsAs1DForOutWhenUnconnected=off
  ao2 : Outport  Port=2  VectorParamsAs1DForOutWhenUnconnected=off
  ao3 : Outport  Port=3  VectorParamsAs1DForOutWhenUnconnected=off
  ao4 : Outport  Port=4  VectorParamsAs1DForOutWhenUnconnected=off
  ai_trigger : Outport  Port=5  VectorParamsAs1DForOutWhenUnconnected=off
  ao_trigger : Outport  Port=6  VectorParamsAs1DForOutWhenUnconnected=off
  cpu_ctrl_monitor : Outport  Port=7  VectorParamsAs1DForOutWhenUnconnected=off
  cpu_ai : Outport  Port=8  VectorParamsAs1DForOutWhenUnconnected=off
  cpu_saturated : Outport  Port=9
  wires:
  Ground5/1 -> DataTypeConversion8/1
  DataTypeConversion8/1 -> ao_trigger/1
  Ground4/1 -> DataTypeConversion7/1
  DataTypeConversion7/1 -> ao4/1
  Ground3/1 -> DataTypeConversion6/1
  DataTypeConversion6/1 -> ao3/1
  Ground2/1 -> DataTypeConversion5/1
  DataTypeConversion5/1 -> ao2/1
  Ground1/1 -> DataTypeConversion4/1
  DataTypeConversion4/1 -> ao1/1
  Ground/1 -> DataTypeConversion3/1
  DataTypeConversion3/1 -> ai_trigger/1
  ai_valid/1 -> Terminator4/1
  ai4/1 -> Terminator3/1
  ai3/1 -> Terminator2/1
  ai2/1 -> Terminator1/1
  ai1/1 -> Terminator/1
  PCIRead_cpu_saturated/1 -> dtc8/1
  dtc8/1 -> DataTypeConversion2/1
  DataTypeConversion2/1 -> cpu_saturated/1
  PCIRead_cpu_ai/1 -> UnPacker/1(packed)
  UnPacker/1(unpacked) -> DataTypeConversion1/1
  DataTypeConversion1/1 -> cpu_ai/1
  PCIRead_cpu_ctrl_monitor/1 -> dtc7/1
  dtc7/1 -> DataTypeConversion/1
  DataTypeConversion/1 -> cpu_ctrl_monitor/1
  dtc6/1 -> PCIWrite_cpu_channel_out/1
  sSpec6/1 -> dtc6/1
  cpu_channel_out/1 -> sSpec6/1
  Packer1/1(packed) -> PCIWrite_cpu_channel_in/1
  cpu_channel_in/1 -> Packer1/1(unpacked)
  dtc5/1 -> PCIWrite_cpu_csr/1
  sSpec5/1 -> dtc5/1
  cpu_csr/1 -> sSpec5/1
  dtc4/1 -> PCIWrite_cpu_gain/1
  sSpec4/1 -> dtc4/1
  cpu_gain/1 -> sSpec4/1
  dtc3/1 -> PCIWrite_cpu_sos2/1
  sSpec3/1 -> dtc3/1
  cpu_sos2/1 -> sSpec3/1
  dtc2/1 -> PCIWrite_cpu_sos1/1
  sSpec2/1 -> dtc2/1
  cpu_sos1/1 -> sSpec2/1
  dtc1/1 -> PCIWrite_ctrl_limit/1
  sSpec1/1 -> dtc1/1
  ctrl_limit/1 -> sSpec1/1
  Packer/1(packed) -> PCIWrite_cpu_ao/1
  cpu_ao/1 -> Packer/1(unpacked)
  dtc/1 -> PCIWrite_cpu_adc_ticks/1
  sSpec/1 -> dtc/1
  cpu_adc_ticks/1 -> sSpec/1

== system SG_library/Source elements/Discrete SOS section DFI serial/Subsystem ==
  trigger : Inport
  Compare To Constant1 : simulink/Logic and Bit Operations/Compare To Constant  relop===  const=12  OutDataTypeStr=boolean
  Constant : Constant  Value=repelem(0:4, 3)  OutMin=0  OutMax=4  OutDataTypeStr=fixdt(0,3,0)  SampleTime=-1
  HDL Counter : hdlsllib/Sources/HDL Counter  CountType=Free running  CountInit=0  CountStep=1  CountMax=4  CountFromType=Initial value  CountFrom=0  CountResetPort=on  CountLoadPort=off  CountEnbPort=on  CountDirPort=off  CountHitOutputPort=off  CountDataType=Unsigned  CountWordLen=8  CountFracLen=0  CountSampTime=-1
  NOT : Logic  Operator=NOT  IconShape=distinctive  AllPortsSameDT=off  OutDataTypeStr=boolean
  Selector : Selector  IndexMode=Zero-based  InputPortWidth=15  IndexOptions=Starting index (port)  Indices=[1 3]  OutputSizes=1
  Unit Delay Enabled Resettable Synchronous : hdlsllib/Discrete/Unit Delay Enabled Resettable Synchronous  InitialCondition=0.0  SampleTime=-1
  count : Outport
  wires:
  HDL Counter/1 -> Compare To Constant1/1, Selector/2
  NOT/1 -> HDL Counter/1
  Selector/1 -> count/1
  Unit Delay Enabled Resettable Synchronous/1 -> NOT/1, HDL Counter/2
  Compare To Constant1/1 -> Unit Delay Enabled Resettable Synchronous/3
  trigger/1 -> Unit Delay Enabled Resettable Synchronous/2, Unit Delay Enabled Resettable Synchronous/1
  Constant/1 -> Selector/1

== system SG_library/Source elements/Generator/gen ==
  note: 0.5[s] rise time
  type : Inport
  Enable : EnablePort  StatesWhenEnabling=reset
  Counter Free-Running : simulink/Sources/Counter Free-Running  NumBits=32  tsamp=ts
  Data Type Conversion : DataTypeConversion  OutDataTypeStr=double  SaturateOnIntegerOverflow=off  RndMeth=Floor
  MATLAB Function : MATLAB Function  TreatAsAtomicUnit=on
  Merge : Merge  Inputs=4
  Signal Specification : SignalSpecification  SampleTime=ts
  Switch Case : SwitchCase  CaseConditions={GeneratorType.rand_white, GeneratorType.rand_pink, GeneratorType.sweep_lin, GeneratorType.sweep_log}  ShowDefaultCase=off
  Switch Case Action Subsystem : Subsystem  TreatAsAtomicUnit=on
  Switch Case Action Subsystem1 : Subsystem  TreatAsAtomicUnit=on
  Switch Case Action Subsystem2 : Subsystem  TreatAsAtomicUnit=on
  Switch Case Action Subsystem3 : Subsystem  TreatAsAtomicUnit=on
  Weighted Sample Time : SampleTimeMath  TsampMathOp=*  weightValue=1
  signal : Outport  OutputWhenDisabled=reset  InitialOutput=0  VectorParamsAs1DForOutWhenUnconnected=off
  wires:
  Counter Free-Running/1 -> Data Type Conversion/1
  MATLAB Function/1(y) -> signal/1
  Weighted Sample Time/1 -> MATLAB Function/2(t)
  Data Type Conversion/1 -> Weighted Sample Time/1
  type/1 -> Switch Case/1
  Signal Specification/1 -> MATLAB Function/1(u)
  Switch Case/1 -> Switch Case Action Subsystem/Action
  Switch Case/2 -> Switch Case Action Subsystem1/Action
  Switch Case/3 -> Switch Case Action Subsystem2/Action
  Switch Case/4 -> Switch Case Action Subsystem3/Action
  Switch Case Action Subsystem/1(Out1) -> Merge/1
  Switch Case Action Subsystem3/1(Out1) -> Merge/4
  Switch Case Action Subsystem1/1(Out1) -> Merge/2
  Switch Case Action Subsystem2/1(Out1) -> Merge/3
  Merge/1 -> Signal Specification/1

== system SG_library/Source elements/SOS filter/Subsystem ==
  u : Inport
  sos : Inport  Port=2
  Reset : ResetPort  DisableCoverage=on  ResetTriggerType=level hold
  Biquad Filter1 : dsparch4/Biquad Filter  FilterSource=Input port(s)  CoeffSource=Specify via dialog  FilterObject=dfilt.df2tsos([1 0.3 0.4],[1 0.1 0.2])  IIRFiltStruct=Direct form II transposed  BiQuadCoeffs=sos1  ScaleValues=1  IC=0  ICnum=0  ICden=0  a0Flag=Error  optimizeScaleValues=on  ScaleValueMode=Assume all are unity and optimize  roundingMode=Floor  overflowMode=off  scaleValueFracLength=14  denProdOutputFracLength=30  denAccumFracLength=30  secondMemoryFracLength=15
  Selector : Selector  NumberOfDimensions=2  InputPortWidth=3  IndexOptions=Select all,Index vector (dialog)  Indices=[1 3],1:3  OutputSizes=1,1
  Selector1 : Selector  NumberOfDimensions=2  InputPortWidth=3  IndexOptions=Select all,Index vector (dialog)  Indices=[1 3],5:6  OutputSizes=1,1
  Transpose : Math  Operator=transpose
  Transpose1 : Math  Operator=transpose
  y : Outport
  wires:
  Transpose/1 -> Biquad Filter1/3
  Biquad Filter1/1 -> y/1
  Selector1/1 -> Transpose/1
  Selector/1 -> Transpose1/1
  Transpose1/1 -> Biquad Filter1/2
  sos/1 -> Selector1/1, Selector/1
  u/1 -> Biquad Filter1/1

== system SG_library/Source elements/SOS filter/Subsystem1 ==
  u : Inport
  sos : Inport  Port=2
  Reset : ResetPort  DisableCoverage=on  ResetTriggerType=level hold
  Biquad Filter1 : dsparch4/Biquad Filter  FilterSource=Input port(s)  CoeffSource=Specify via dialog  FilterObject=dfilt.df2tsos([1 0.3 0.4],[1 0.1 0.2])  IIRFiltStruct=Direct form II transposed  BiQuadCoeffs=sos1  ScaleValues=1  IC=0  ICnum=0  ICden=0  a0Flag=Error  optimizeScaleValues=on  ScaleValueMode=Assume all are unity and optimize  roundingMode=Floor  overflowMode=off  scaleValueFracLength=14  denProdOutputFracLength=30  denAccumFracLength=30  secondMemoryFracLength=15
  Selector : Selector  NumberOfDimensions=2  InputPortWidth=3  IndexOptions=Select all,Index vector (dialog)  Indices=[1 3],1:3  OutputSizes=1,1
  Selector1 : Selector  NumberOfDimensions=2  InputPortWidth=3  IndexOptions=Select all,Index vector (dialog)  Indices=[1 3],5:6  OutputSizes=1,1
  Transpose : Math  Operator=transpose
  Transpose1 : Math  Operator=transpose
  y : Outport
  wires:
  Transpose/1 -> Biquad Filter1/3
  Biquad Filter1/1 -> y/1
  Selector1/1 -> Transpose/1
  Selector/1 -> Transpose1/1
  Transpose1/1 -> Biquad Filter1/2
  sos/1 -> Selector1/1, Selector/1
  u/1 -> Biquad Filter1/1
